simulink model "saab93_combustion"  (R2018a)
settings: Solver=VariableStepDiscrete  StartTime=0.0  StopTime=1220  RelTol=1e-3  EnableMultiTasking=on
undefined symbols (not defined in the file): DiscIntNeverNeededParam, h, H_u, k_cs, rho_f
libraries: qss_tb_library x5
settings Model: Creator=grauers  LastModifiedBy=Luís Miranda
settings DataIOCC: LimitDataPoints=on  SaveFormat=Array  SignalLoggingSaveFormat=ModelDataLogs
settings OptimizationCC: InitFltsAndDblsToZero=on  LifeSpan=inf
settings DebuggingCC: SaveWithParameterizedLinksMsg=none  UnderspecifiedInitializationDetection=Classic  MergeDetectMultiDrivingBlocksExec=none  SignalResolutionControl=TryResolveAllWithWarning  SolverPrmCheckMsg=warning  MultiTaskDSMMsg=warning  MultiTaskCondExecSysMsg=none  FcnCallInpInsideContextMsg=warning  SFUnexpectedBacktrackingDiag=warning  SFNoUnconditionalDefaultTransitionDiag=warning  SFExecutionAtInitializationDiag=none
settings HardwareCC: ProdBitPerPointer=32  ProdBitPerSizeT=32  ProdBitPerPtrDiffT=32  ProdLargestAtomicFloat=None  ProdIntDivRoundTo=Undefined  ProdEndianess=Unspecified  ProdWordSize=32  ProdHWDeviceType=32-bit Generic
settings ModelReferenceCC: PropagateSignalLabelsOutOfModel=off
settings CodeAppCC: StateflowObjectComments=on
settings GRTTargetCC: TargetFcnLib=ansi_tfl_tmw.mat  TargetLangStandard=C89/C90 (ANSI)  CombineOutputUpdateFcns=off  GRTInterface=on
settings ConfigComp: CovMetricSettings=dw  CovHtmlReporting=on  CovSaveCumulativeToWorkspaceVar=on  CovSaveSingleToWorkspaceVar=on  CovExternalEMLEnable=off

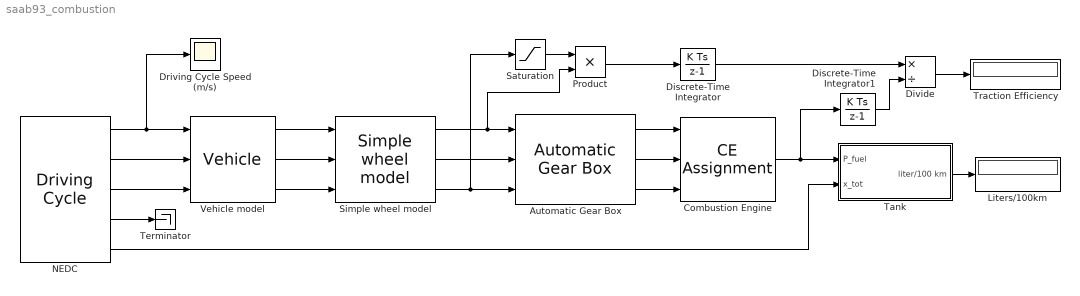
== system saab93_combustion ==
  "Automatic Gear Box " : qss_tb_library/Gear System/Automatic Gear Box  Tag=transmission  nog=5  i=[3.38 1.76 1.12 0.89 0.7]  i_diff=4.45  gearon=[10 25 40 70]  gearoff=[2 15 30 50]  d=0.62  e_GT=0.98  P_GT0=300  w_wheel_min=1
  Combustion Engine : qss_tb_library/Energy Converter/CE Assignment  Tag=combustion engine  engine_type=Gasoline  P_ice=95  ENABLE_FUEL_CUTOFF=off
  Discrete-Time Integrator : DiscreteIntegrator  SampleTime=-1  ICPrevOutput=DiscIntNeverNeededParam  ICPrevScaledInput=DiscIntNeverNeededParam
  Discrete-Time Integrator1 : DiscreteIntegrator  SampleTime=-1  ICPrevOutput=DiscIntNeverNeededParam  ICPrevScaledInput=DiscIntNeverNeededParam
  Divide : Product  Inputs=*/
  Driving Cycle Speed (m/s) : Scope
  Liters/100km : Display
  NEDC : qss_tb_library/Driving Cycle/Driving Cycle  Tag=cycle  cyclename1=NEDC  stepsize=1  autostop=on
  Product : Product
  Saturation : Saturate  UpperLimit=100000  LowerLimit=0
  "Simple wheel model " : qss_tb_library/Vehicle/Simple wheel model  Tag=simple transmission  d_wheel=0.62
  Tank : Subsystem  Tag=tank  mask(Tank){fuel=Gasoline, flag_cold_start=off}
      mask prompts: flag_cold_start "Include cold start losses"
      mask help:
      | This block integrates the power (the fuel mass flow) required by the combustion engine or the fuel cell and calculates the energy consumption in liter/100 km.
      |
      | Input:
      | =====
      | 	P_fuel	Power (fuel mass flow) required [W]
      | 	x_tot	Total distance [m]
      |
      | Output:
      | ======
      | 	V	Fuel consumption [liter/100 km]
      mask init:
      | init_tank;
      mask TypeOptions fuel: Gasoline | Diesel | Hydrogen
  Terminator : Terminator
  Traction Efficiency : Display
  Vehicle model : qss_tb_library/Vehicle/Vehicle  Tag=vehicle  m_f=1295+80+100  A_f=2  cw=0.30  mu=0.013  k_inertia=4
  wires:
  Vehicle model/1 -> "Simple wheel model "/1
  Vehicle model/2 -> "Simple wheel model "/2
  Vehicle model/3 -> "Simple wheel model "/3
  "Automatic Gear Box "/1 -> Combustion Engine/1
  "Automatic Gear Box "/2 -> Combustion Engine/2
  "Automatic Gear Box "/3 -> Combustion Engine/3
  Tank/1(liter/100 km) -> Liters/100km/1
  Combustion Engine/1 -> Discrete-Time Integrator1/1, Tank/1(P_fuel)
  NEDC/5 -> Tank/2(x_tot)
  NEDC/1 -> Vehicle model/1, Driving Cycle Speed (m/s)/1
  NEDC/3 -> Vehicle model/3
  NEDC/4 -> Terminator/1
  "Simple wheel model "/1 -> Product/2, "Automatic Gear Box "/1
  "Simple wheel model "/2 -> "Automatic Gear Box "/2
  "Simple wheel model "/3 -> "Automatic Gear Box "/3, Saturation/1
  Saturation/1 -> Product/1
  Product/1 -> Discrete-Time Integrator/1
  Discrete-Time Integrator/1 -> Divide/1
  Discrete-Time Integrator1/1 -> Divide/2
  Divide/1 -> Traction Efficiency/1
  NEDC/2 -> Vehicle model/2

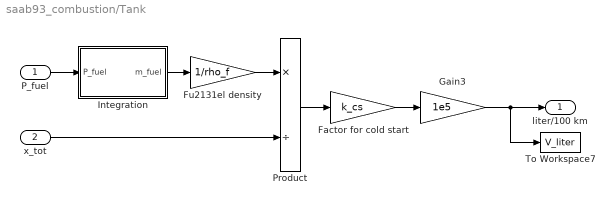
== system saab93_combustion/Tank ==
  P_fuel : Inport
  x_tot : Inport  Port=2
  Factor for cold start : Gain  Gain=k_cs  SaturateOnIntegerOverflow=on  OutDataTypeStr=Inherit: Same as input  ParamDataTypeStr=Inherit: Same as input
  Fu2131el density : Gain  Gain=1/rho_f  SaturateOnIntegerOverflow=on  OutDataTypeStr=Inherit: Same as input  ParamDataTypeStr=Inherit: Same as input
  Gain3 : Gain  Gain=1e5  SaturateOnIntegerOverflow=on  OutDataTypeStr=Inherit: Same as input  ParamDataTypeStr=Inherit: Same as input
  Integration : Subsystem
  Product : Product  Inputs=*/  SaturateOnIntegerOverflow=on  RndMeth=Zero  InputSameDT=on  OutDataTypeStr=Inherit: Same as first input
  To Workspace7 : ToWorkspace  VariableName=V_liter  SampleTime=-1
  liter/100 km : Outport  InitialOutput=0
  wires:
  Factor for cold start/1 -> Gain3/1
  Product/1 -> Factor for cold start/1
  Fu2131el density/1 -> Product/1
  Gain3/1 -> To Workspace7/1, liter/100 km/1
  Integration/1(m_fuel) -> Fu2131el density/1
  x_tot/1 -> Product/2
  P_fuel/1 -> Integration/1(P_fuel)

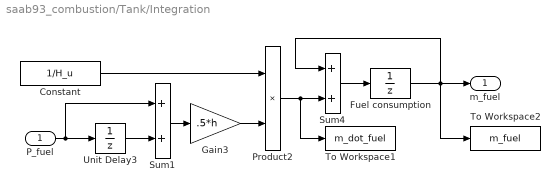
== system saab93_combustion/Tank/Integration ==
  P_fuel : Inport
  Constant : Constant  Value=1/H_u
  Fuel consumption : UnitDelay  SampleTime=h
  Gain3 : Gain  Gain=.5*h  SaturateOnIntegerOverflow=on  OutDataTypeStr=Inherit: Same as input  ParamDataTypeStr=Inherit: Same as input
  Product2 : Product  SaturateOnIntegerOverflow=on  RndMeth=Zero  InputSameDT=on  OutDataTypeStr=Inherit: Same as first input
  Sum1 : Sum  SaturateOnIntegerOverflow=on  InputSameDT=on  OutDataTypeStr=Inherit: Same as first input
  Sum4 : Sum  SaturateOnIntegerOverflow=on  InputSameDT=on  OutDataTypeStr=Inherit: Same as first input
  To Workspace1 : ToWorkspace  VariableName=m_dot_fuel  SampleTime=-1
  To Workspace2 : ToWorkspace  VariableName=m_fuel  SampleTime=-1
  Unit Delay3 : UnitDelay  SampleTime=h
  m_fuel : Outport  InitialOutput=0
  wires:
  Product2/1 -> To Workspace1/1, Sum4/2
  Sum4/1 -> Fuel consumption/1
  Fuel consumption/1 -> To Workspace2/1, Sum4/1, m_fuel/1
  Sum1/1 -> Gain3/1
  Unit Delay3/1 -> Sum1/2
  P_fuel/1 -> Unit Delay3/1, Sum1/1
  Gain3/1 -> Product2/2
  Constant/1 -> Product2/1
